simulink model "Motor_Cable_verification"  (R2019b)
settings: Solver=VariableStepAuto  StartTime=0.0  StopTime=10.0  RelTol=1e-3
undefined symbols (not defined in the file): d_drum, p, theta_m
settings Model: Creator=zceeash  LastModifiedBy=arund

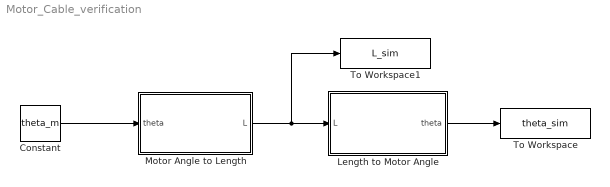
== system Motor_Cable_verification ==
  Constant : Constant  Value=theta_m
  Length to Motor Angle : Subsystem
  Motor Angle to Length : Subsystem
  To Workspace : ToWorkspace  VariableName=theta_sim  SaveFormat=Timeseries  SampleTime=-1
  To Workspace1 : ToWorkspace  VariableName=L_sim  SaveFormat=Timeseries  SampleTime=-1
  wires:
  Motor Angle to Length/1(L) -> To Workspace1/1, Length to Motor Angle/1(L)
  Constant/1 -> Motor Angle to Length/1(theta)
  Length to Motor Angle/1(theta) -> To Workspace/1

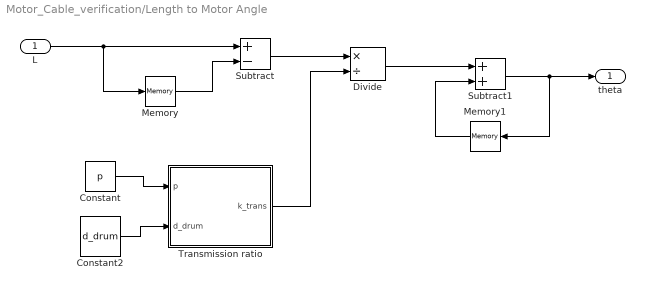
== system Motor_Cable_verification/Length to Motor Angle ==
  L : Inport
  Constant : Constant  Value=p
  Constant2 : Constant  Value=d_drum
  Divide : Product  Inputs=*/
  Memory : Memory
  Memory1 : Memory
  Subtract : Sum  Inputs=+-
  Subtract1 : Sum
  Transmission ratio : Subsystem
  theta : Outport
  wires:
  Memory/1 -> Subtract/2
  Memory1/1 -> Subtract1/2
  Subtract1/1 -> Memory1/1, theta/1
  Subtract/1 -> Divide/1
  Divide/1 -> Subtract1/1
  L/1 -> Subtract/1, Memory/1
  Constant/1 -> Transmission ratio/1(p)
  Constant2/1 -> Transmission ratio/2(d_drum)
  Transmission ratio/1(k_trans) -> Divide/2

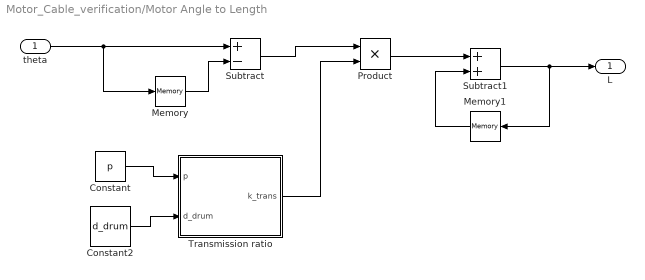
== system Motor_Cable_verification/Motor Angle to Length ==
  theta : Inport
  Constant : Constant  Value=p
  Constant2 : Constant  Value=d_drum
  Memory : Memory
  Memory1 : Memory
  Product : Product
  Subtract : Sum  Inputs=+-
  Subtract1 : Sum
  Transmission ratio : Subsystem
  L : Outport
  wires:
  theta/1 -> Subtract/1, Memory/1
  Memory/1 -> Subtract/2
  Product/1 -> Subtract1/1
  Memory1/1 -> Subtract1/2
  Subtract1/1 -> Memory1/1, L/1
  Subtract/1 -> Product/1
  Constant/1 -> Transmission ratio/1(p)
  Transmission ratio/1(k_trans) -> Product/2
  Constant2/1 -> Transmission ratio/2(d_drum)

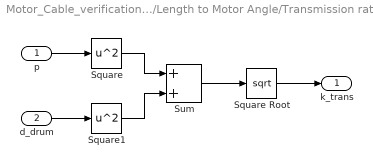
== system Motor_Cable_verification/Length to Motor Angle/Transmission ratio ==
  p : Inport
  d_drum : Inport  Port=2
  Square : Math  Operator=square  SignedPower=off  SaturateOnIntegerOverflow=on
  Square Root : Sqrt  SaturateOnIntegerOverflow=on
  Square1 : Math  Operator=square  SignedPower=off  SaturateOnIntegerOverflow=on
  Sum : Sum
  k_trans : Outport
  wires:
  Square/1 -> Sum/1
  p/1 -> Square/1
  d_drum/1 -> Square1/1
  Square1/1 -> Sum/2
  Sum/1 -> Square Root/1
  Square Root/1 -> k_trans/1

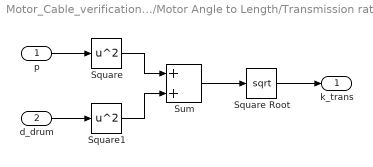
== system Motor_Cable_verification/Motor Angle to Length/Transmission ratio ==
  p : Inport
  d_drum : Inport  Port=2
  Square : Math  Operator=square  SignedPower=off  SaturateOnIntegerOverflow=on
  Square Root : Sqrt  SaturateOnIntegerOverflow=on
  Square1 : Math  Operator=square  SignedPower=off  SaturateOnIntegerOverflow=on
  Sum : Sum
  k_trans : Outport
  wires:
  Square/1 -> Sum/1
  p/1 -> Square/1
  d_drum/1 -> Square1/1
  Square1/1 -> Sum/2
  Sum/1 -> Square Root/1
  Square Root/1 -> k_trans/1
